simulink subsystem "sub_encoder_velocidad_R"  (R2023b)
settings: Solver=VariableStepAuto  StartTime=0.0  StopTime=10.0  RelTol=1e-3
libraries: arduinosensorlib x2, simulink x1
settings Model: Creator=ricfe  LastModifiedBy=ricfe

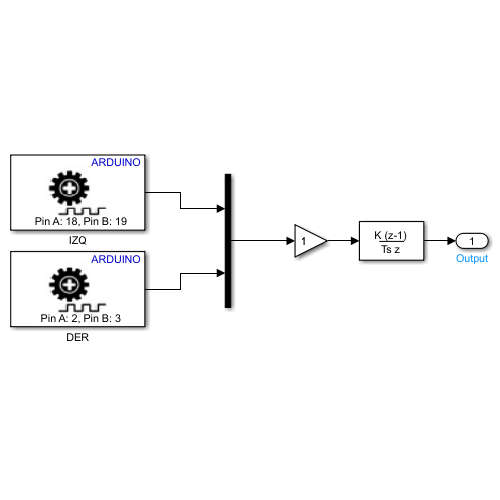
[thumbnail: Simulink's stored preview of the top-level diagram]
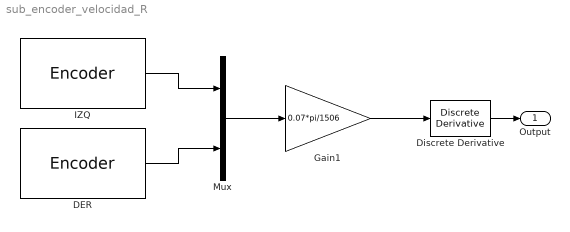
== system sub_encoder_velocidad_R ==
  DER : arduinosensorlib/Encoder  InputA=2  InputB=3  Mode=No reset  SampleTime=-1
  Discrete Derivative : simulink/Discrete/Discrete Derivative  gainval=1.0  ICPrevScaledInput=0.0  OutMin=[]  OutMax=[]  OutDataType=fixdt(1, 16)  OutScaling=2^-10  DoSatur=off
  Gain1 : Gain  Gain=0.07*pi/1506  ParamDataTypeStr=double
  IZQ : arduinosensorlib/Encoder  InputA=18  InputB=19  Mode=No reset  SampleTime=-1
  Mux : Mux  Inputs=2
  Output : Outport
  wires:
  DER/1 -> Mux/2
  IZQ/1 -> Mux/1
  Mux/1 -> Gain1/1
  Gain1/1 -> Discrete Derivative/1
  Discrete Derivative/1 -> Output/1
